simulink model "va_circuit"  (R2025b)
settings: Solver=VariableStepAuto  StartTime=0  StopTime=1  RelTol=1e-3
values from neighbouring files (symbols this model uses):
  fs = 96000    [create_trainset.m]    (also in solveCircuit.m = 1/(t(2)-t(1)))
libraries: fl_lib x3, nesl_utility x3
settings DataIOCC: OutputOption=SpecifiedOutputTimes  OutputTimes=[0;1.04166666666667e-05;2.08333333333333e-05;3.125e-05;4.16666666666667e-05;5.20833333333333e-05;6.25e-05;7.29166666666667e-05;8.33333333333333e-05;9.375e-05;0.000104166666666667;0.000114583333333333;0.000125;0.000135416666666667;0.000145833333333333;0.00015625;0.000166666666666667;0.000177083333333333;0.0001875;0.000197916666666667;0.000208333333333333;0.00021875;0.000229166666666667;0.000239583333333333;0.00025;0.000260416666666667;0.000270833333333333;0.00028125;0.000291666666666667;0.000302083333333333;0.0003125;0.000322916666666667;0.000333333333333333;0.00034375;0.000354166666666667;0.000364583333333333;0.000375;0.000385416666666667;0.000395833333333333;0.00040625;0.000416666666666667;0.000427083333333333;0.0004375;0.000447916666666667;0.000458333333333333;0.00046875;0.000479166666666667;0.000489583333333333;0.0005;0.000510416666666667;0.000520833333333333;0.00053125;0.000541666666666667;0.000552083333333333;0.0005625;0.000572916666666667;0.000583333333333333;0.00059375;0.000604166666666667;0.000614583333333333;0.000625;0.000635416666666667;0.000645833333333333;0.00065625;0.000666666666666667;0.000677083333333333;0.0006875;0.000697916666666667;0.000708333333333333;0.00071875;0.000729166666666667;0.000739583333333333;0.00075;0.000760416666666667;0.000770833333333333;0.00078125;0.000791666666666667;0.000802083333333333;0.0008125;0.000822916666666667;0.000833333333333333;0.00084375;0.000854166666666667;0.000864583333333333;0.000875;0.000885416666666667;0.000895833333333333;0.00090625;0.000916666666666667;0.000927083333333333;0.0009375;0.000947916666666667;0.000958333333333333;0.00096875;0.000979166666666667;0.000989583333333333;0.001;0.00101041666666667;0.00102083333333333;0.00103125;0.00104166666666667;0.00105208333333333;0.0010625;0.00107291666666667;0.00108333333333333;0.00109375;0.00110416666666667;0.00111458333333333;0.001125;0.00113541666666667;0.00114583333333333;0.00115625;0.00116666666666667;0.00117708333333333;0.0011875;0.00119791666666667;0.00120833333333333;0.00121875;0.00122916666666667;0.00123958333333333;0.00125;0.00126041666666667;0.00127083333333333;0.00128125;0.00129166666666667;0.00130208333333333;0.0013125;0.00132291666666667;0.00133333333333333;0.00134375;0.00135416666666667;0.00136458333333333;0.001375;0.00138541666666667;0.00139583333333333;0.00140625;0.00141666666666667;0.00142708333333333;0.0014375;0.00144791666666667;0.00145833333333333;0.00146875;0.00147916666666667;0.00148958333333333;0.0015;0.00151041666666667;0.00152083333333333;0.00153125;0.00154166666666667;0.00155208333333333;0.0015625;0.00157291666666667;0.00158333333333333;0.00159375;0.00160416666666667;0.00161458333333333;0.001625;0.00163541666666667;0.00164583333333333;0.00165625;0.00166666666666667;0.00167708333333333;0.0016875;0.00169791666666667;0.00170833333333333;0.00171875;0.00172916666666667;0.00173958333333333;0.00175;0.00176041666666667;0.00177083333333333;0.00178125;0.00179166666666667;0.00180208333333333;0.0018125;0.00182291666666667;0.00183333333333333;0.00184375;0.00185416666666667;0.00186458333333333;0.001875;0.00188541666666667;0.00189583333333333;0.00190625;0.00191666666666667;0.00192708333333333;0.0019375;0.00194791666666667;0.00195833333333333;0.00196875;0.00197916666666667;0.00198958333333333;0.002;0.00201041666666667;0.00202083333333333;0.00203125;0.00204166666666667;0.00205208333333333;0.0020625;0.00207291666666667;0.00208333333333333;0.00209375;0.00210416666666667;0.00211458333333333;0.002125;0.00213541666666667;0.00214583333333333;0.00215625;0.00216666666666667;0.00217708333333333;0.0021875;0.00219791666666667;0.00220833333333333;0.00221875;0.00222916666666667;0.00223958333333333;0.00225;0.00226041666666667;0.00227083333333333;0.00228125;0.00229166666666667;0.00230208333333333;0.0023125;0.00232291666666667;0.00233333333333333;0.00234375;0.00235416666666667;0.00236458333333333;0.002375;0.00238541666666667;0.00239583333333333;0.00240625;0.00241666666666667;0.00242708333333333;0.0024375;0.00244791666666667 ...(+1476003 chars)]

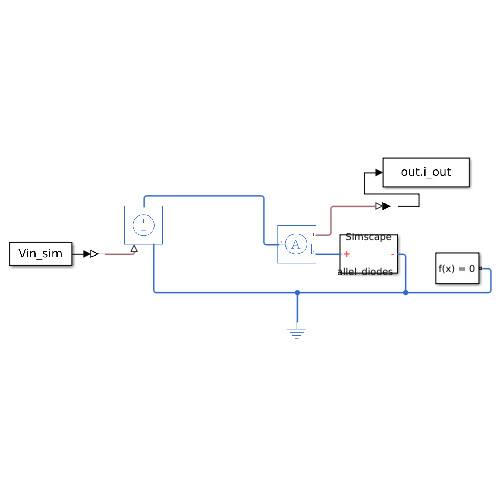
[thumbnail: Simulink's stored preview of the top-level diagram]
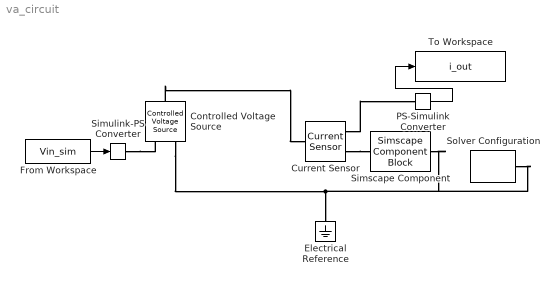
== system va_circuit ==
  Controlled Voltage Source : fl_lib/Electrical/Electrical Sources/Controlled Voltage Source
  Current Sensor : fl_lib/Electrical/Electrical Sensors/Current Sensor
  Electrical Reference : fl_lib/Electrical/Electrical Elements/Electrical Reference
  From Workspace : FromWorkspace  VariableName=Vin_sim
  PS-Simulink Converter : nesl_utility/PS-Simulink Converter  PhysicalDomain=network_engine_domain  SubClassName=ps_output  LeftPortType=input  RightPortType=output  PseudoPeriodic=off  Frequencies=[]  VectorFormat=inherit  Unit=A  AffineConversion=on
  Simscape Component : SimscapeComponentBlock  SourceFile=antiparallel_diodes_1n4148  ComponentPath=antiparallel_diodes_1n4148  ComponentVariants="[\"antiparallel_diodes_1n4148\"]"  ComponentVariantNames="[\"antiparallel_diodes_1n4148\"]"  ClassName=antiparallel_diodes_1n4148  SchemaVersion=1  Is=2.52e-9 A  Rs=0.568 Ohm  eta=1.752  Vt=25.85e-3 V  Rp=1e8 Ohm  i_specify=off  i_priority=None  i=0 A  i_nominal_specify=off  i_nominal_value=1  i_nominal_unit=A  v_specify=off  v_priority=None  v=0 V  v_nominal_specify=off  v_nominal_value=1  v_nominal_unit=V  i_fwd_specify=off  i_fwd_priority=None  i_fwd=0 A  i_fwd_nominal_specify=off  i_fwd_nominal_value=1  i_fwd_nominal_unit=A  i_rev_specify=off  i_rev_priority=None  i_rev=0 A  i_rev_nominal_specify=off  i_rev_nominal_value=1  i_rev_nominal_unit=A
      settings: CopyFcn=simscape.sscblock.internal.componentBlockCallback(gcbh,'COPY')  PreCopyFcn=simscape.sscblock.internal.componentBlockCallback(gcbh,'PRECOPY')  PreDeleteFcn=simscape.sscblock.internal.componentBlockCallback(gcbh,'PREDELETE')  InternalSimscapePortConfiguration="{\"Bottom\":[],\"Left\":[{\"id\":\"p\",\"label\":\"+\",\"type\":\"foundation.electrical.electrical\"}],\"Right\":[{\"id\":\"n\",\"label\":\"-\",\"type\":\"foundation.electrical.electrical\"}],\"Top\":[]}"
      mask Type: Antiparallel 1N4148 Diode Pair
  Simulink-PS Converter : nesl_utility/Simulink-PS Converter  PhysicalDomain=network_engine_domain  SubClassName=ps_input  LeftPortType=input  RightPortType=output  PseudoPeriodic=off  Frequencies=[]  NoiseDistribution=none  NoiseParameters=[]  Unit=V  AffineConversion=on  FilteringAndDerivatives=provide  SimscapeFilterOrder=1  InputFilterTimeConstant=0.001  UdotUserProvided=0
  Solver Configuration : nesl_utility/Solver Configuration  PhysicalDomain=network_engine_domain  SubClassName=solver  LeftPortType=input  RightPortType=generic  Tones=[]  Harmonics=[]  SimulateNoise=off  Profile=off  UseLocalSampling=off  EnableSwitchedLinearOptims=on  FrequencyDomain=off  UseCCode=off  RelTol=0.001  AbsTol=0.001  MinStep=1e-09  ToWorkspace=off  RevertToSquareIcSolve=off  NumHomotopyIterations=100  PhasorMode=off  PhasorModeNumHarmonics=1  ConsistencySolver=NEWTON_XTOL_AFTER_FTOL  IndexReductionMethod=DerivativeReplacement  DoDC=off  ResidualTolerance=1e-09  ConsistencyTolSource=GLOBAL  ConsistencyAbsTol=0.001  ConsistencyRelTol=0.001  ConsistencyTolFactor=0.001  UseLocalSolver=off  LocalSolverChoice=NE_BACKWARD_EULER_ADVANCER  ResolveIndetEquations=on  FunctionEvalNumThread=1  LocalSolverSampleTime=1/fs  DoFixedCost=off  MaxNonlinIter=3  MaxModeIter=2  ComputeImpulses=off  ImpulseIterations=2  LinearAlgebra=Full  LinearAlgebraNumThread=0  EquationFormulation=NE_TIME_EF  DelaysMemoryBudget=1024  AutomaticFiltering=on  FilteringTimeConstant=0.001  PartitionStorageMethod=AS_NEEDED  PartitionMemoryBudget=1024  PartitionMethod=ROBUST  MultibodyUseLocalSolver=off  MultibodyLocalSolverChoice=ODE1  MultibodyLocalSolverSampleTime=0.001
  To Workspace : ToWorkspace  VariableName=i_out  SampleTime=-1
  wires:
  From Workspace/1 -> Simulink-PS Converter/1
  PS-Simulink Converter/1 -> To Workspace/1
  connections:
  Simulink-PS Converter/RConn1 -- Controlled Voltage Source/RConn1
  Current Sensor/RConn1 -- PS-Simulink Converter/LConn1
  Controlled Voltage Source/RConn2 -- Simscape Component/RConn1 -- Solver Configuration/RConn1 -- Electrical Reference/LConn1
  Controlled Voltage Source/LConn1 -- Current Sensor/LConn1
  Current Sensor/RConn2 -- Simscape Component/LConn1
